simulink model "gm_moving_avg"  (R2020a)
settings: Solver=FixedStepDiscrete  StartTime=0.0  StopTime=0.5  RelTol=1e-3
settings Model: Creator=sumee  LastModifiedBy=sumee
settings OptimizationCC: BlockReduction=off  ConditionallyExecuteInputs=off
settings DebuggingCC: InheritedTsInSrcMsg=none

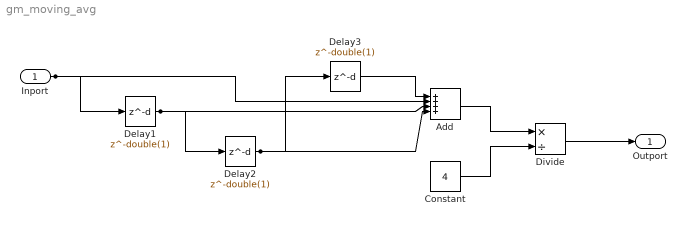
== system gm_moving_avg ==
  Inport : Inport  OutDataTypeStr=fixdt(1, 32, 16)  PortDimensions=1  SampleTime=6.1096312226594e-08
  Add : Sum  Inputs=++++  AccumDataTypeStr=fixdt(1, 32, 16)  OutDataTypeStr=fixdt(1, 32, 16)  SampleTime=6.1096312226594e-08
  Constant : Constant  Value=4  OutDataTypeStr=int16
  Delay1 : Delay  DelayLength=double(1)  InitialCondition=0  SampleTime=6.1096312226594e-08
  Delay2 : Delay  DelayLength=double(1)  InitialCondition=0  SampleTime=6.1096312226594e-08
  Delay3 : Delay  DelayLength=double(1)  InitialCondition=0  SampleTime=6.1096312226594e-08
  Divide : Product  Inputs=*/  OutDataTypeStr=fixdt(1, 32, 16)  RndMeth=Zero  SaturateOnIntegerOverflow=on  SampleTime=6.1096312226594e-08
  Outport : Outport  OutDataTypeStr=fixdt(1,32,16)  PortDimensions=1
  wires:
  Inport/1 -> Add/2, Delay1/1
  Add/1 -> Divide/1
  Constant/1 -> Divide/2
  Delay1/1 -> Add/3, Delay2/1
  Delay2/1 -> Add/4, Delay3/1
  Delay3/1 -> Add/1
  Divide/1 -> Outport/1
